simulink model "q_four_aw"  (R2019b)
settings: Solver=VariableStepAuto  StartTime=0.0  StopTime=5  RelTol=1e-3
values from neighbouring files (symbols this model uses):
  A_fs = [-0.5 0 -455;0 -2.9 455; 1 -1 0]    [ex4.m]    (also in ex5.m; ex5test.m)
  B_fs = [17 0; 0 -5; 0 0]    [ex4.m]    (also in ex5.m; ex5test.m)
  C_fs = [1 0 0; 0 1 0; 0 0 1]    [ex4.m]    (also in ex5.m; ex5test.m)
  D_fs = [0 0;0 0; 0 0]    [ex4.m]    (also in ex5.m; ex5test.m)
  kq4 = place(A4, B4, p4)    [ex4.m]    (also in ex5.m; ex5test.m)
settings Model: Creator=kecy6rkk  LastModifiedBy=rafek
settings SFSimCC: CustomCodeUndefinedFunction=UseInterfaceOnly

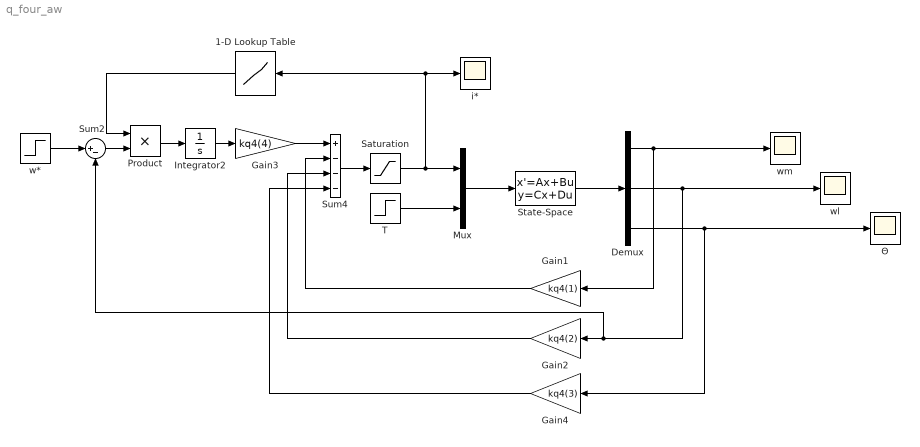
== system q_four_aw ==
  1-D Lookup Table : Lookup_n-D  NumberOfTableDimensions=1  BreakpointsForDimension1=[-100, -42, -41.9, 0, 41.9, 42, 100]  Table=[0, 0, 1, 1, 1, 0, 0]  InternalRulePriority=Speed  RndMeth=Simplest  InputSameDT=on
  Demux : Demux  Outputs=3
  Gain1 : Gain  Gain=kq4(1)
  Gain2 : Gain  Gain=kq4(2)
  Gain3 : Gain  Gain=kq4(4)
  Gain4 : Gain  Gain=kq4(3)
  Integrator2 : Integrator
  Mux : Mux  Inputs=2
  Product : Product
  Saturation : Saturate  UpperLimit=42  LowerLimit=-42
  State-Space : StateSpace  A=A_fs  B=B_fs  C=C_fs  D=D_fs  InitialCondition=0
  Sum2 : Sum  Inputs=|+-
  Sum4 : Sum  Inputs=+---
  T : Step  Time=0  After=75  SampleTime=0
  i* : Scope
  w* : Step  Time=0  After=100  SampleTime=0
  wl : Scope
  wm : Scope
  Θ : Scope
  wires:
  Mux/1 -> State-Space/1
  State-Space/1 -> Demux/1
  Gain1/1 -> Sum4/2
  Demux/3 -> Gain4/1, Θ/1
  T/1 -> Mux/2
  Integrator2/1 -> Gain3/1
  Demux/1 -> Gain1/1, wm/1
  Gain4/1 -> Sum4/4
  w*/1 -> Sum2/1
  Gain3/1 -> Sum4/1
  Gain2/1 -> Sum4/3
  Demux/2 -> Sum2/2, Gain2/1, wl/1
  Product/1 -> Integrator2/1
  Sum2/1 -> Product/2
  1-D Lookup Table/1 -> Product/1
  Sum4/1 -> Saturation/1
  Saturation/1 -> i*/1, 1-D Lookup Table/1, Mux/1
